simulink model "ControladoresLibro"  (R2025b)
settings: Solver=VariableStepAuto  StartTime=0.0  StopTime=10.0  RelTol=1e-3
libraries: fl_lib x33, slpidlib x18, nesl_utility x18, ee_lib x6
settings Model: Creator=Usuario  LastModifiedBy=Usuario

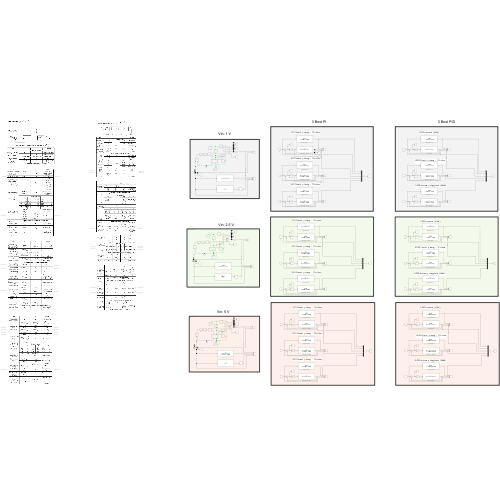
[thumbnail: Simulink's stored preview of the top-level diagram]
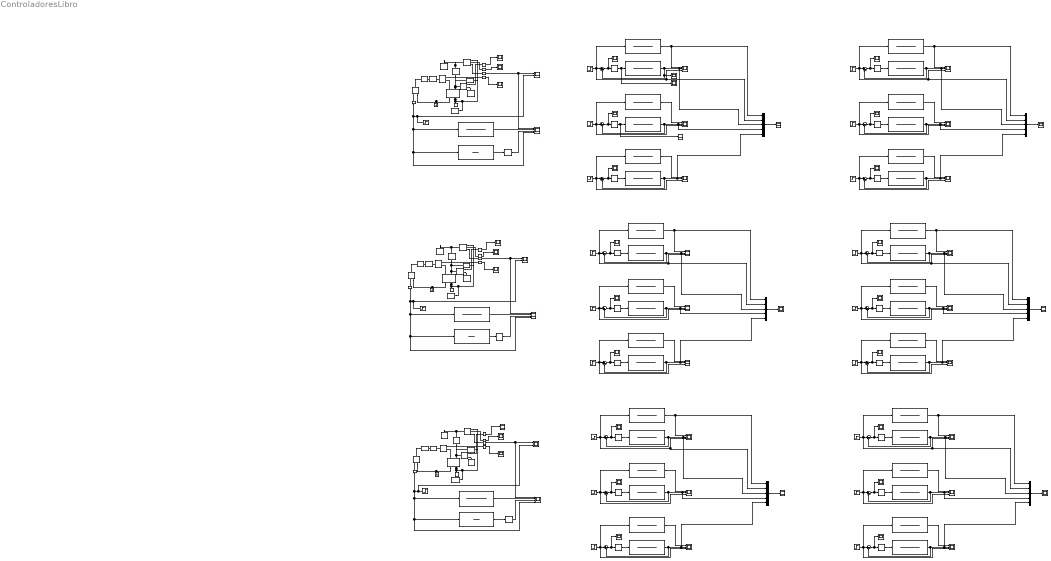
== system ControladoresLibro ==
  note: Voltaje Entrada 1V
  note: --------->
  note: thetha_l
  note: Vin
  note: --------->
  note: Ia
  note: Voltaje Entrada 5V
  note: Vin
  note: thetha_l
  note: Ia
  note: Vin
  note: --------->
  note: Ia
  note: --------->
  note: 1-PI Cluett y Wang - TCL=6tm
  note: <---------
  note: --------->
  note: <---------
  note: 3-PI Cluett y Wang - TCL=4tm
  note: 2-PID Cluett y Wang - TCL=6tm
  note: <---------
  note: thetha_l
  note: 2-PID Cluett y Wang - TCL=6tm
  note: 2-PID Cluett y Wang - TCL=6tm
  note: --------->
  note: 1-PID Leonard (1994)
  note: 3 Best PID
  note: <---------
  note: Vin: 2.5 V
  note: <---------
  note: --------->
  note: 3-PI Cluett y Wang - TCL=4tm
  note: <---------
  note: <---------
  note: <---------
  note: <---------
  note: <---------
  note: --------->
  note: 3-PI Cluett y Wang - TCL=4tm
  note: --------->
  note: 3-PID Astrom y Hagglund (2006)
  note: 2-PI Cluett y Wang - TCL=5tm
  note: --------->
  note: 2-PI Cluett y Wang - TCL=5tm
  note: <---------
  note: 3 Best PI
  note: --------->
  note: 1-PID Leonard (1994)
  note: <---------
  note: 3-PID Astrom y Hagglund (2006)
  note: 2-PI Cluett y Wang - TCL=5tm
  note: Vin: 5 V
  note: 1-PI Cluett y Wang - TCL=6tm
  note: <---------
  note: <---------
  note: --------->
  note: 1-PID Leonard (1994)
  note: --------->
  note: Vin: 1 V
  note: 3-PID Astrom y Hagglund (2006)
  note: <---------
  note: <---------
  note: <---------
  note: <---------
  note: --------->
  note: --------->
  note: 1-PI Cluett y Wang - TCL=6tm
  note: --------->
  note: --------->
  note: Voltaje Entrada 2.5V
  Astrom y Hagglund : TransferFcn  Numerator=[33792]  Denominator=[1 2500 55822 0]
  Astrom y Hagglund1 : TransferFcn  Numerator=[33792]  Denominator=[1 2500 55822 0]
  Astrom y Hagglund2 : TransferFcn  Numerator=[33792]  Denominator=[1 2500 55822 0]
  Cluett y Wang - TCL=4tm : TransferFcn  Numerator=[33792]  Denominator=[1 2500 55822 0]
  Cluett y Wang - TCL=4tm1 : TransferFcn  Numerator=[33792]  Denominator=[1 2500 55822 0]
  Cluett y Wang - TCL=4tm2 : TransferFcn  Numerator=[33792]  Denominator=[1 2500 55822 0]
  Cluett y Wang - TCL=5tm : TransferFcn  Numerator=[33792]  Denominator=[1 2500 55822 0]
  Cluett y Wang - TCL=5tm1 : TransferFcn  Numerator=[33792]  Denominator=[1 2500 55822 0]
  Cluett y Wang - TCL=5tm2 : TransferFcn  Numerator=[33792]  Denominator=[1 2500 55822 0]
  Cluett y Wang - TCL=6tm{,1..5} (6 alike) : TransferFcn  Numerator=[33792]  Denominator=[1 2500 55822 0]
  Controlled Voltage Source : fl_lib/Electrical/Electrical Sources/Controlled Voltage Source
  Controlled Voltage Source1 : fl_lib/Electrical/Electrical Sources/Controlled Voltage Source
  Controlled Voltage Source2 : fl_lib/Electrical/Electrical Sources/Controlled Voltage Source
  Current Sensor : fl_lib/Electrical/Electrical Sensors/Current Sensor
  Current Sensor1 : fl_lib/Electrical/Electrical Sensors/Current Sensor
  Current Sensor2 : fl_lib/Electrical/Electrical Sensors/Current Sensor
  Dm : fl_lib/Mechanical/Rotational Elements/Rotational Damper  D=2.5e-7 N*m*s/rad  w_specify=off  w_priority=None  w=0 rad/s  w_nominal_specify=off  w_nominal_value=1  w_nominal_unit=rad/s  t_specify=off  t_priority=None  t=0 N*m  t_nominal_specify=off  t_nominal_value=1  t_nominal_unit=N*m
  Dm1 : fl_lib/Mechanical/Rotational Elements/Rotational Damper  D=2.5e-7 N*m*s/rad  w_specify=off  w_priority=None  w=0 rad/s  w_nominal_specify=off  w_nominal_value=1  w_nominal_unit=rad/s  t_specify=off  t_priority=None  t=0 N*m  t_nominal_specify=off  t_nominal_value=1  t_nominal_unit=N*m
  Dm2 : fl_lib/Mechanical/Rotational Elements/Rotational Damper  D=2.5e-7 N*m*s/rad  w_specify=off  w_priority=None  w=0 rad/s  w_nominal_specify=off  w_nominal_value=1  w_nominal_unit=rad/s  t_specify=off  t_priority=None  t=0 N*m  t_nominal_specify=off  t_nominal_value=1  t_nominal_unit=N*m
  Electrical Reference : fl_lib/Electrical/Electrical Elements/Electrical Reference
  Electrical Reference1 : fl_lib/Electrical/Electrical Elements/Electrical Reference
  Electrical Reference2 : fl_lib/Electrical/Electrical Elements/Electrical Reference
  Gear Box : fl_lib/Mechanical/Mechanisms/Gear Box  ratio=1/275.6923  t_in_specify=off  t_in_priority=None  t_in=0 N*m  t_in_nominal_specify=off  t_in_nominal_value=1  t_in_nominal_unit=N*m  t_out_specify=off  t_out_priority=None  t_out=0 N*m  t_out_nominal_specify=off  t_out_nominal_value=1  t_out_nominal_unit=N*m
  Gear Box1 : fl_lib/Mechanical/Mechanisms/Gear Box  ratio=1/275.6923  t_in_specify=off  t_in_priority=None  t_in=0 N*m  t_in_nominal_specify=off  t_in_nominal_value=1  t_in_nominal_unit=N*m  t_out_specify=off  t_out_priority=None  t_out=0 N*m  t_out_nominal_specify=off  t_out_nominal_value=1  t_out_nominal_unit=N*m
  Gear Box2 : fl_lib/Mechanical/Mechanisms/Gear Box  ratio=1/275.6923  t_in_specify=off  t_in_priority=None  t_in=0 N*m  t_in_nominal_specify=off  t_in_nominal_value=1  t_in_nominal_unit=N*m  t_out_specify=off  t_out_priority=None  t_out=0 N*m  t_out_nominal_specify=off  t_out_nominal_value=1  t_out_nominal_unit=N*m
  Ideal Rotational Motion Sensor : fl_lib/Mechanical/Mechanical Sensors/Ideal Rotational Motion Sensor  reference=foundation.enum.MeasurementReference.difference  acceleration_port=false  velocity_port=true  position_port=true  wrap_angle=false  offset=0 rad
  Ideal Rotational Motion Sensor1 : fl_lib/Mechanical/Mechanical Sensors/Ideal Rotational Motion Sensor  reference=foundation.enum.MeasurementReference.difference  acceleration_port=false  velocity_port=true  position_port=true  wrap_angle=false  offset=0 rad
  Ideal Rotational Motion Sensor2 : fl_lib/Mechanical/Mechanical Sensors/Ideal Rotational Motion Sensor  reference=foundation.enum.MeasurementReference.difference  acceleration_port=false  velocity_port=true  position_port=true  wrap_angle=false  offset=0 rad
  Ideal Torque Sensor1 : fl_lib/Mechanical/Mechanical Sensors/Ideal Torque Sensor
  Ideal Torque Sensor2 : fl_lib/Mechanical/Mechanical Sensors/Ideal Torque Sensor
  Ideal Torque Sensor3 : fl_lib/Mechanical/Mechanical Sensors/Ideal Torque Sensor
  In1 : Step  SampleTime=0
  In2 : Step  After=2.5  SampleTime=0
  In3 : Step  After=5  SampleTime=0
  In4 : Step  SampleTime=0
  In5 : Step  After=2.5  SampleTime=0
  In6 : Step  After=5  SampleTime=0
  Jl : fl_lib/Mechanical/Rotational Elements/Inertia  inertia=2e-6 kg*m^2  num_ports=foundation.enum.numPorts2.one  w_specify=off  w_priority=High  w=0 rad/s  w_nominal_specify=off  w_nominal_value=1  w_nominal_unit=rad/s  t_specify=off  t_priority=None  t=0 N*m  t_nominal_specify=off  t_nominal_value=1  t_nominal_unit=N*m
  Jl1 : fl_lib/Mechanical/Rotational Elements/Inertia  inertia=2e-6 kg*m^2  num_ports=foundation.enum.numPorts2.one  w_specify=off  w_priority=High  w=0 rad/s  w_nominal_specify=off  w_nominal_value=1  w_nominal_unit=rad/s  t_specify=off  t_priority=None  t=0 N*m  t_nominal_specify=off  t_nominal_value=1  t_nominal_unit=N*m
  Jl2 : fl_lib/Mechanical/Rotational Elements/Inertia  inertia=2e-6 kg*m^2  num_ports=foundation.enum.numPorts2.one  w_specify=off  w_priority=High  w=0 rad/s  w_nominal_specify=off  w_nominal_value=1  w_nominal_unit=rad/s  t_specify=off  t_priority=None  t=0 N*m  t_nominal_specify=off  t_nominal_value=1  t_nominal_unit=N*m
  Jm : fl_lib/Mechanical/Rotational Elements/Inertia  inertia=6.3173e-7 kg*m^2  num_ports=foundation.enum.numPorts2.one  w_specify=off  w_priority=High  w=0 rad/s  w_nominal_specify=off  w_nominal_value=1  w_nominal_unit=rad/s  t_specify=off  t_priority=None  t=0 N*m  t_nominal_specify=off  t_nominal_value=1  t_nominal_unit=N*m
  Jm1 : fl_lib/Mechanical/Rotational Elements/Inertia  inertia=6.3173e-7 kg*m^2  num_ports=foundation.enum.numPorts2.one  w_specify=off  w_priority=High  w=0 rad/s  w_nominal_specify=off  w_nominal_value=1  w_nominal_unit=rad/s  t_specify=off  t_priority=None  t=0 N*m  t_nominal_specify=off  t_nominal_value=1  t_nominal_unit=N*m
  Jm2 : fl_lib/Mechanical/Rotational Elements/Inertia  inertia=6.3173e-7 kg*m^2  num_ports=foundation.enum.numPorts2.one  w_specify=off  w_priority=High  w=0 rad/s  w_nominal_specify=off  w_nominal_value=1  w_nominal_unit=rad/s  t_specify=off  t_priority=None  t=0 N*m  t_nominal_specify=off  t_nominal_value=1  t_nominal_unit=N*m
  L : ee_lib/Passive/Inductor  l=1 mH  enable_L_tol=ee.enum.toleranceApplication.none  L_tol=20  tol_distribution=ee.enum.toleranceDistribution.uniform  nSigma=4  r=0 Ohm  g=0 1/Ohm  enable_operating_limits=ee.enum.enable.no  operating_limit_action=ee.enum.passive.reportOpLim.warn  max_working_current=1 A  power_rating=1 W  i_L_specify=off  i_L_priority=High  i_L=0 A  i_L_nominal_specify=off  i_L_nominal_value=1  i_L_nominal_unit=A
  L1 : ee_lib/Passive/Inductor  l=1 mH  enable_L_tol=ee.enum.toleranceApplication.none  L_tol=20  tol_distribution=ee.enum.toleranceDistribution.uniform  nSigma=4  r=0 Ohm  g=0 1/Ohm  enable_operating_limits=ee.enum.enable.no  operating_limit_action=ee.enum.passive.reportOpLim.warn  max_working_current=1 A  power_rating=1 W  i_L_specify=off  i_L_priority=High  i_L=0 A  i_L_nominal_specify=off  i_L_nominal_value=1  i_L_nominal_unit=A
  L2 : ee_lib/Passive/Inductor  l=1 mH  enable_L_tol=ee.enum.toleranceApplication.none  L_tol=20  tol_distribution=ee.enum.toleranceDistribution.uniform  nSigma=4  r=0 Ohm  g=0 1/Ohm  enable_operating_limits=ee.enum.enable.no  operating_limit_action=ee.enum.passive.reportOpLim.warn  max_working_current=1 A  power_rating=1 W  i_L_specify=off  i_L_priority=High  i_L=0 A  i_L_nominal_specify=off  i_L_nominal_value=1  i_L_nominal_unit=A
  Leonard (1994) : TransferFcn  Numerator=[33792]  Denominator=[1 2500 55822 0]
  Leonard (1994)1 : TransferFcn  Numerator=[33792]  Denominator=[1 2500 55822 0]
  Leonard (1994)2 : TransferFcn  Numerator=[33792]  Denominator=[1 2500 55822 0]
  Mechanical Rotational Reference : fl_lib/Mechanical/Rotational Elements/Mechanical Rotational Reference
  Mechanical Rotational Reference1 : fl_lib/Mechanical/Rotational Elements/Mechanical Rotational Reference
  Mechanical Rotational Reference2 : fl_lib/Mechanical/Rotational Elements/Mechanical Rotational Reference
  Mux{1..6} (6 alike) : Mux  Inputs=5
  Original Function {1..18} (18 alike) : TransferFcn  Numerator=[33792]  Denominator=[1 2500 55822 0]
  PID Controller{7,10,12,15,17} (5 alike) : slpidlib/PID Controller  Controller=PI  Form=Parallel  TimeDomain=Continuous-time  UseExternalTs=off  SampleTime=-1  IntegratorMethod=Forward Euler  FilterMethod=Forward Euler  ControllerParametersSource=internal  P=11.1080  I=21.4441  UseKiTs=off  D=1.316  UseExternalDerivativeSource=off  N=100  UseFilter=on  TunerSelectOption=Transfer Function Based (PID Tuner App)  InitialConditionSource=internal  InitialConditionForIntegrator=0  InitialConditionForFilter=0  DifferentiatorICPrevScaledInput=0  ExternalReset=none  TrackingMode=off  Kt=1  LimitOutput=off  SatLimitsSource=internal  UpperSaturationLimit=inf  LowerSaturationLimit=-inf  LinearizeAsGain=on  AntiWindupMode=none  Kb=1  LimitIntegrator=off  UpperIntegratorSaturationLimit=inf  LowerIntegratorSaturationLimit=-inf  POutMin=[]  POutMax=[]  IOutMin=[]  IOutMax=[]  DOutMin=[]  DOutMax=[]  NOutMin=[]  NOutMax=[]  SumOutMin=[]  SumOutMax=[]  SaturationOutMin=[]  SaturationOutMax=[]  PParamMin=[]  PParamMax=[]  IParamMin=[]  IParamMax=[]  DParamMin=[]  DParamMax=[]  NParamMin=[]  NParamMax=[]  KbParamMin=[]  KbParamMax=[]  KtParamMin=[]  KtParamMax=[]  KbOutMin=[]  KbOutMax=[]  KtOutMin=[]  KtOutMax=[]  IntegratorOutMin=[]  IntegratorOutMax=[]  FilterOutMin=[]  FilterOutMax=[]  SumI1OutMin=[]  SumI1OutMax=[]  SumI2OutMin=[]  SumI2OutMax=[]  SumI3OutMin=[]  SumI3OutMax=[]  SumI4OutMin=[]  SumI4OutMax=[]  SumDOutMin=[]  SumDOutMax=[]  DifferentiatorOutMin=[]  DifferentiatorOutMax=[]  FilterDiffOutCoefMin=[]  FilterDiffOutCoefMax=[]  ReciprocalOutMin=[]  ReciprocalOutMax=[]  SumDenOutMin=[]  SumDenOutMax=[]  SumNumOutMin=[]  SumNumOutMax=[]  DivideOutMin=[]  DivideOutMax=[]  UdiffTsProdOutMin=[]  UdiffTsProdOutMax=[]  NTsProdOutMin=[]  NTsProdOutMax=[]  UintegralTsProdOutMin=[]  UintegralTsProdOutMax=[]  UngainTsProdOutMin=[]  UngainTsProdOutMax=[]  ClampingZeroOutDataTypeStr=Inherit: Inherit via back propagation  ClampingZeroOutMin=[]  ClampingZeroOutMax=[]  FilterDenConstantOutDataTypeStr=Inherit: Inherit via back propagation  FilterDenConstantOutMin=[]  FilterDenConstantOutMax=[]  PCopyOutDataTypeStr=Inherit: Inherit via back propagation  PCopyOutMin=[]  PCopyOutMax=[]  NCopyOutDataTypeStr=Inherit: Inherit via back propagation  NCopyOutMin=[]  NCopyOutMax=[]  IntegratorContinuousStateAttributes=''  IntegratorStateMustResolveToSignalObject=off  IntegratorRTWStateStorageClass=Auto  FilterContinuousStateAttributes=''  FilterStateMustResolveToSignalObject=off  FilterRTWStateStorageClass=Auto  ParallelPVariant=InternalParameters  IdealPVariant=Disabled  IVariant=InternalParameters  DVariant=Disabled  IntegratorVariant=Continuous  SatVariant=Disabled  AWVariant=Passthrough  PCopyVariant=Disabled  TRVariant=Disabled  FdbkBlocksVariant=Forward  IdealPFdbkVariant=Disabled  SatFdbkVariant=Disabled  DerivativeFilterVariant=Disabled  NVariant=Disabled  NCopyVariant=Disabled_SignalSpec  FilterICVariant=Disabled  IntegratorICVariant=InternalICs  ExternalResetVariant=Disabled  TRSumVariant=Passthrough  SumFdbkVariant=Disabled  SumVariant=Sum_PI  TsampFilterVariant=InternalTs  TsampNgainVariant=Passthrough  TsampIntegralVariant=Disabled_SignalSpec  ExternalSaturationOutDataTypeStr=Inherit: Same as second input  DerivativeSourceVariant=Disabled  PreIntVariant=InternalPreInt
  PID Controller{8,11,13,16,18} (5 alike) : slpidlib/PID Controller  Controller=PI  Form=Parallel  TimeDomain=Continuous-time  UseExternalTs=off  SampleTime=-1  IntegratorMethod=Forward Euler  FilterMethod=Forward Euler  ControllerParametersSource=internal  P=13.2561  I=31.0787  UseKiTs=off  D=1.316  UseExternalDerivativeSource=off  N=100  UseFilter=on  TunerSelectOption=Transfer Function Based (PID Tuner App)  InitialConditionSource=internal  InitialConditionForIntegrator=0  InitialConditionForFilter=0  DifferentiatorICPrevScaledInput=0  ExternalReset=none  TrackingMode=off  Kt=1  LimitOutput=off  SatLimitsSource=internal  UpperSaturationLimit=inf  LowerSaturationLimit=-inf  LinearizeAsGain=on  AntiWindupMode=none  Kb=1  LimitIntegrator=off  UpperIntegratorSaturationLimit=inf  LowerIntegratorSaturationLimit=-inf  POutMin=[]  POutMax=[]  IOutMin=[]  IOutMax=[]  DOutMin=[]  DOutMax=[]  NOutMin=[]  NOutMax=[]  SumOutMin=[]  SumOutMax=[]  SaturationOutMin=[]  SaturationOutMax=[]  PParamMin=[]  PParamMax=[]  IParamMin=[]  IParamMax=[]  DParamMin=[]  DParamMax=[]  NParamMin=[]  NParamMax=[]  KbParamMin=[]  KbParamMax=[]  KtParamMin=[]  KtParamMax=[]  KbOutMin=[]  KbOutMax=[]  KtOutMin=[]  KtOutMax=[]  IntegratorOutMin=[]  IntegratorOutMax=[]  FilterOutMin=[]  FilterOutMax=[]  SumI1OutMin=[]  SumI1OutMax=[]  SumI2OutMin=[]  SumI2OutMax=[]  SumI3OutMin=[]  SumI3OutMax=[]  SumI4OutMin=[]  SumI4OutMax=[]  SumDOutMin=[]  SumDOutMax=[]  DifferentiatorOutMin=[]  DifferentiatorOutMax=[]  FilterDiffOutCoefMin=[]  FilterDiffOutCoefMax=[]  ReciprocalOutMin=[]  ReciprocalOutMax=[]  SumDenOutMin=[]  SumDenOutMax=[]  SumNumOutMin=[]  SumNumOutMax=[]  DivideOutMin=[]  DivideOutMax=[]  UdiffTsProdOutMin=[]  UdiffTsProdOutMax=[]  NTsProdOutMin=[]  NTsProdOutMax=[]  UintegralTsProdOutMin=[]  UintegralTsProdOutMax=[]  UngainTsProdOutMin=[]  UngainTsProdOutMax=[]  ClampingZeroOutDataTypeStr=Inherit: Inherit via back propagation  ClampingZeroOutMin=[]  ClampingZeroOutMax=[]  FilterDenConstantOutDataTypeStr=Inherit: Inherit via back propagation  FilterDenConstantOutMin=[]  FilterDenConstantOutMax=[]  PCopyOutDataTypeStr=Inherit: Inherit via back propagation  PCopyOutMin=[]  PCopyOutMax=[]  NCopyOutDataTypeStr=Inherit: Inherit via back propagation  NCopyOutMin=[]  NCopyOutMax=[]  IntegratorContinuousStateAttributes=''  IntegratorStateMustResolveToSignalObject=off  IntegratorRTWStateStorageClass=Auto  FilterContinuousStateAttributes=''  FilterStateMustResolveToSignalObject=off  FilterRTWStateStorageClass=Auto  ParallelPVariant=InternalParameters  IdealPVariant=Disabled  IVariant=InternalParameters  DVariant=Disabled  IntegratorVariant=Continuous  SatVariant=Disabled  AWVariant=Passthrough  PCopyVariant=Disabled  TRVariant=Disabled  FdbkBlocksVariant=Forward  IdealPFdbkVariant=Disabled  SatFdbkVariant=Disabled  DerivativeFilterVariant=Disabled  NVariant=Disabled  NCopyVariant=Disabled_SignalSpec  FilterICVariant=Disabled  IntegratorICVariant=InternalICs  ExternalResetVariant=Disabled  TRSumVariant=Passthrough  SumFdbkVariant=Disabled  SumVariant=Sum_PI  TsampFilterVariant=InternalTs  TsampNgainVariant=Passthrough  TsampIntegralVariant=Disabled_SignalSpec  ExternalSaturationOutDataTypeStr=Inherit: Same as second input  DerivativeSourceVariant=Disabled  PreIntVariant=InternalPreInt
  PID Controller{6,9,14,19,23} (5 alike) : slpidlib/PID Controller  Controller=PI  Form=Parallel  TimeDomain=Continuous-time  UseExternalTs=off  SampleTime=-1  IntegratorMethod=Forward Euler  FilterMethod=Forward Euler  ControllerParametersSource=internal  P=9.5711  I=15.6962  UseKiTs=off  D=1.316  UseExternalDerivativeSource=off  N=100  UseFilter=on  TunerSelectOption=Transfer Function Based (PID Tuner App)  InitialConditionSource=internal  InitialConditionForIntegrator=0  InitialConditionForFilter=0  DifferentiatorICPrevScaledInput=0  ExternalReset=none  TrackingMode=off  Kt=1  LimitOutput=off  SatLimitsSource=internal  UpperSaturationLimit=inf  LowerSaturationLimit=-inf  LinearizeAsGain=on  AntiWindupMode=none  Kb=1  LimitIntegrator=off  UpperIntegratorSaturationLimit=inf  LowerIntegratorSaturationLimit=-inf  POutMin=[]  POutMax=[]  IOutMin=[]  IOutMax=[]  DOutMin=[]  DOutMax=[]  NOutMin=[]  NOutMax=[]  SumOutMin=[]  SumOutMax=[]  SaturationOutMin=[]  SaturationOutMax=[]  PParamMin=[]  PParamMax=[]  IParamMin=[]  IParamMax=[]  DParamMin=[]  DParamMax=[]  NParamMin=[]  NParamMax=[]  KbParamMin=[]  KbParamMax=[]  KtParamMin=[]  KtParamMax=[]  KbOutMin=[]  KbOutMax=[]  KtOutMin=[]  KtOutMax=[]  IntegratorOutMin=[]  IntegratorOutMax=[]  FilterOutMin=[]  FilterOutMax=[]  SumI1OutMin=[]  SumI1OutMax=[]  SumI2OutMin=[]  SumI2OutMax=[]  SumI3OutMin=[]  SumI3OutMax=[]  SumI4OutMin=[]  SumI4OutMax=[]  SumDOutMin=[]  SumDOutMax=[]  DifferentiatorOutMin=[]  DifferentiatorOutMax=[]  FilterDiffOutCoefMin=[]  FilterDiffOutCoefMax=[]  ReciprocalOutMin=[]  ReciprocalOutMax=[]  SumDenOutMin=[]  SumDenOutMax=[]  SumNumOutMin=[]  SumNumOutMax=[]  DivideOutMin=[]  DivideOutMax=[]  UdiffTsProdOutMin=[]  UdiffTsProdOutMax=[]  NTsProdOutMin=[]  NTsProdOutMax=[]  UintegralTsProdOutMin=[]  UintegralTsProdOutMax=[]  UngainTsProdOutMin=[]  UngainTsProdOutMax=[]  ClampingZeroOutDataTypeStr=Inherit: Inherit via back propagation  ClampingZeroOutMin=[]  ClampingZeroOutMax=[]  FilterDenConstantOutDataTypeStr=Inherit: Inherit via back propagation  FilterDenConstantOutMin=[]  FilterDenConstantOutMax=[]  PCopyOutDataTypeStr=Inherit: Inherit via back propagation  PCopyOutMin=[]  PCopyOutMax=[]  NCopyOutDataTypeStr=Inherit: Inherit via back propagation  NCopyOutMin=[]  NCopyOutMax=[]  IntegratorContinuousStateAttributes=''  IntegratorStateMustResolveToSignalObject=off  IntegratorRTWStateStorageClass=Auto  FilterContinuousStateAttributes=''  FilterStateMustResolveToSignalObject=off  FilterRTWStateStorageClass=Auto  ParallelPVariant=InternalParameters  IdealPVariant=Disabled  IVariant=InternalParameters  DVariant=Disabled  IntegratorVariant=Continuous  SatVariant=Disabled  AWVariant=Passthrough  PCopyVariant=Disabled  TRVariant=Disabled  FdbkBlocksVariant=Forward  IdealPFdbkVariant=Disabled  SatFdbkVariant=Disabled  DerivativeFilterVariant=Disabled  NVariant=Disabled  NCopyVariant=Disabled_SignalSpec  FilterICVariant=Disabled  IntegratorICVariant=InternalICs  ExternalResetVariant=Disabled  TRSumVariant=Passthrough  SumFdbkVariant=Disabled  SumVariant=Sum_PI  TsampFilterVariant=InternalTs  TsampNgainVariant=Passthrough  TsampIntegralVariant=Disabled_SignalSpec  ExternalSaturationOutDataTypeStr=Inherit: Same as second input  DerivativeSourceVariant=Disabled  PreIntVariant=InternalPreInt
  PID Controller20 : slpidlib/PID Controller  Controller=PID  Form=Parallel  TimeDomain=Continuous-time  UseExternalTs=off  SampleTime=-1  IntegratorMethod=Forward Euler  FilterMethod=Forward Euler  ControllerParametersSource=internal  P=26.1447  I=46.1855  UseKiTs=off  D=0.4974  UseExternalDerivativeSource=off  N=100  UseFilter=on  TunerSelectOption=Transfer Function Based (PID Tuner App)  InitialConditionSource=internal  InitialConditionForIntegrator=0  InitialConditionForFilter=0  DifferentiatorICPrevScaledInput=0  ExternalReset=none  TrackingMode=off  Kt=1  LimitOutput=off  SatLimitsSource=internal  UpperSaturationLimit=inf  LowerSaturationLimit=-inf  LinearizeAsGain=on  AntiWindupMode=none  Kb=1  LimitIntegrator=off  UpperIntegratorSaturationLimit=inf  LowerIntegratorSaturationLimit=-inf  POutMin=[]  POutMax=[]  IOutMin=[]  IOutMax=[]  DOutMin=[]  DOutMax=[]  NOutMin=[]  NOutMax=[]  SumOutMin=[]  SumOutMax=[]  SaturationOutMin=[]  SaturationOutMax=[]  PParamMin=[]  PParamMax=[]  IParamMin=[]  IParamMax=[]  DParamMin=[]  DParamMax=[]  NParamMin=[]  NParamMax=[]  KbParamMin=[]  KbParamMax=[]  KtParamMin=[]  KtParamMax=[]  KbOutMin=[]  KbOutMax=[]  KtOutMin=[]  KtOutMax=[]  IntegratorOutMin=[]  IntegratorOutMax=[]  FilterOutMin=[]  FilterOutMax=[]  SumI1OutMin=[]  SumI1OutMax=[]  SumI2OutMin=[]  SumI2OutMax=[]  SumI3OutMin=[]  SumI3OutMax=[]  SumI4OutMin=[]  SumI4OutMax=[]  SumDOutMin=[]  SumDOutMax=[]  DifferentiatorOutMin=[]  DifferentiatorOutMax=[]  FilterDiffOutCoefMin=[]  FilterDiffOutCoefMax=[]  ReciprocalOutMin=[]  ReciprocalOutMax=[]  SumDenOutMin=[]  SumDenOutMax=[]  SumNumOutMin=[]  SumNumOutMax=[]  DivideOutMin=[]  DivideOutMax=[]  UdiffTsProdOutMin=[]  UdiffTsProdOutMax=[]  NTsProdOutMin=[]  NTsProdOutMax=[]  UintegralTsProdOutMin=[]  UintegralTsProdOutMax=[]  UngainTsProdOutMin=[]  UngainTsProdOutMax=[]  ClampingZeroOutDataTypeStr=Inherit: Inherit via back propagation  ClampingZeroOutMin=[]  ClampingZeroOutMax=[]  FilterDenConstantOutDataTypeStr=Inherit: Inherit via back propagation  FilterDenConstantOutMin=[]  FilterDenConstantOutMax=[]  PCopyOutDataTypeStr=Inherit: Inherit via back propagation  PCopyOutMin=[]  PCopyOutMax=[]  NCopyOutDataTypeStr=Inherit: Inherit via back propagation  NCopyOutMin=[]  NCopyOutMax=[]  IntegratorContinuousStateAttributes=''  IntegratorStateMustResolveToSignalObject=off  IntegratorRTWStateStorageClass=Auto  FilterContinuousStateAttributes=''  FilterStateMustResolveToSignalObject=off  FilterRTWStateStorageClass=Auto  ParallelPVariant=InternalParameters  IdealPVariant=Disabled  IVariant=InternalParameters  DVariant=InternalParameters  IntegratorVariant=Continuous  SatVariant=Disabled  AWVariant=Passthrough  PCopyVariant=Disabled  TRVariant=Disabled  FdbkBlocksVariant=Forward  IdealPFdbkVariant=Disabled  SatFdbkVariant=Disabled  DerivativeFilterVariant=ContFilter  NVariant=InternalParameters  NCopyVariant=Disabled  FilterICVariant=InternalICsFilter  IntegratorICVariant=InternalICs  ExternalResetVariant=Disabled  TRSumVariant=Passthrough  SumFdbkVariant=Disabled  SumVariant=Sum_PID  TsampFilterVariant=InternalTs  TsampNgainVariant=Passthrough  TsampIntegralVariant=Disabled_SignalSpec  ExternalSaturationOutDataTypeStr=Inherit: Same as second input  DerivativeSourceVariant=ErrorSignal  PreIntVariant=InternalPreInt
  PID Controller21 : slpidlib/PID Controller  Controller=PID  Form=Parallel  TimeDomain=Continuous-time  UseExternalTs=off  SampleTime=-1  IntegratorMethod=Forward Euler  FilterMethod=Forward Euler  ControllerParametersSource=internal  P=9.5711  I=15.6962  UseKiTs=off  D=0.0564  UseExternalDerivativeSource=off  N=100  UseFilter=on  TunerSelectOption=Transfer Function Based (PID Tuner App)  InitialConditionSource=internal  InitialConditionForIntegrator=0  InitialConditionForFilter=0  DifferentiatorICPrevScaledInput=0  ExternalReset=none  TrackingMode=off  Kt=1  LimitOutput=off  SatLimitsSource=internal  UpperSaturationLimit=inf  LowerSaturationLimit=-inf  LinearizeAsGain=on  AntiWindupMode=none  Kb=1  LimitIntegrator=off  UpperIntegratorSaturationLimit=inf  LowerIntegratorSaturationLimit=-inf  POutMin=[]  POutMax=[]  IOutMin=[]  IOutMax=[]  DOutMin=[]  DOutMax=[]  NOutMin=[]  NOutMax=[]  SumOutMin=[]  SumOutMax=[]  SaturationOutMin=[]  SaturationOutMax=[]  PParamMin=[]  PParamMax=[]  IParamMin=[]  IParamMax=[]  DParamMin=[]  DParamMax=[]  NParamMin=[]  NParamMax=[]  KbParamMin=[]  KbParamMax=[]  KtParamMin=[]  KtParamMax=[]  KbOutMin=[]  KbOutMax=[]  KtOutMin=[]  KtOutMax=[]  IntegratorOutMin=[]  IntegratorOutMax=[]  FilterOutMin=[]  FilterOutMax=[]  SumI1OutMin=[]  SumI1OutMax=[]  SumI2OutMin=[]  SumI2OutMax=[]  SumI3OutMin=[]  SumI3OutMax=[]  SumI4OutMin=[]  SumI4OutMax=[]  SumDOutMin=[]  SumDOutMax=[]  DifferentiatorOutMin=[]  DifferentiatorOutMax=[]  FilterDiffOutCoefMin=[]  FilterDiffOutCoefMax=[]  ReciprocalOutMin=[]  ReciprocalOutMax=[]  SumDenOutMin=[]  SumDenOutMax=[]  SumNumOutMin=[]  SumNumOutMax=[]  DivideOutMin=[]  DivideOutMax=[]  UdiffTsProdOutMin=[]  UdiffTsProdOutMax=[]  NTsProdOutMin=[]  NTsProdOutMax=[]  UintegralTsProdOutMin=[]  UintegralTsProdOutMax=[]  UngainTsProdOutMin=[]  UngainTsProdOutMax=[]  ClampingZeroOutDataTypeStr=Inherit: Inherit via back propagation  ClampingZeroOutMin=[]  ClampingZeroOutMax=[]  FilterDenConstantOutDataTypeStr=Inherit: Inherit via back propagation  FilterDenConstantOutMin=[]  FilterDenConstantOutMax=[]  PCopyOutDataTypeStr=Inherit: Inherit via back propagation  PCopyOutMin=[]  PCopyOutMax=[]  NCopyOutDataTypeStr=Inherit: Inherit via back propagation  NCopyOutMin=[]  NCopyOutMax=[]  IntegratorContinuousStateAttributes=''  IntegratorStateMustResolveToSignalObject=off  IntegratorRTWStateStorageClass=Auto  FilterContinuousStateAttributes=''  FilterStateMustResolveToSignalObject=off  FilterRTWStateStorageClass=Auto  ParallelPVariant=InternalParameters  IdealPVariant=Disabled  IVariant=InternalParameters  DVariant=InternalParameters  IntegratorVariant=Continuous  SatVariant=Disabled  AWVariant=Passthrough  PCopyVariant=Disabled  TRVariant=Disabled  FdbkBlocksVariant=Forward  IdealPFdbkVariant=Disabled  SatFdbkVariant=Disabled  DerivativeFilterVariant=ContFilter  NVariant=InternalParameters  NCopyVariant=Disabled  FilterICVariant=InternalICsFilter  IntegratorICVariant=InternalICs  ExternalResetVariant=Disabled  TRSumVariant=Passthrough  SumFdbkVariant=Disabled  SumVariant=Sum_PID  TsampFilterVariant=InternalTs  TsampNgainVariant=Passthrough  TsampIntegralVariant=Disabled_SignalSpec  ExternalSaturationOutDataTypeStr=Inherit: Same as second input  DerivativeSourceVariant=ErrorSignal  PreIntVariant=InternalPreInt
  PID Controller22 : slpidlib/PID Controller  Controller=PID  Form=Parallel  TimeDomain=Continuous-time  UseExternalTs=off  SampleTime=-1  IntegratorMethod=Forward Euler  FilterMethod=Forward Euler  ControllerParametersSource=internal  P=15.8988  I=42.8309  UseKiTs=off  D=0.3689  UseExternalDerivativeSource=off  N=100  UseFilter=on  TunerSelectOption=Transfer Function Based (PID Tuner App)  InitialConditionSource=internal  InitialConditionForIntegrator=0  InitialConditionForFilter=0  DifferentiatorICPrevScaledInput=0  ExternalReset=none  TrackingMode=off  Kt=1  LimitOutput=off  SatLimitsSource=internal  UpperSaturationLimit=inf  LowerSaturationLimit=-inf  LinearizeAsGain=on  AntiWindupMode=none  Kb=1  LimitIntegrator=off  UpperIntegratorSaturationLimit=inf  LowerIntegratorSaturationLimit=-inf  POutMin=[]  POutMax=[]  IOutMin=[]  IOutMax=[]  DOutMin=[]  DOutMax=[]  NOutMin=[]  NOutMax=[]  SumOutMin=[]  SumOutMax=[]  SaturationOutMin=[]  SaturationOutMax=[]  PParamMin=[]  PParamMax=[]  IParamMin=[]  IParamMax=[]  DParamMin=[]  DParamMax=[]  NParamMin=[]  NParamMax=[]  KbParamMin=[]  KbParamMax=[]  KtParamMin=[]  KtParamMax=[]  KbOutMin=[]  KbOutMax=[]  KtOutMin=[]  KtOutMax=[]  IntegratorOutMin=[]  IntegratorOutMax=[]  FilterOutMin=[]  FilterOutMax=[]  SumI1OutMin=[]  SumI1OutMax=[]  SumI2OutMin=[]  SumI2OutMax=[]  SumI3OutMin=[]  SumI3OutMax=[]  SumI4OutMin=[]  SumI4OutMax=[]  SumDOutMin=[]  SumDOutMax=[]  DifferentiatorOutMin=[]  DifferentiatorOutMax=[]  FilterDiffOutCoefMin=[]  FilterDiffOutCoefMax=[]  ReciprocalOutMin=[]  ReciprocalOutMax=[]  SumDenOutMin=[]  SumDenOutMax=[]  SumNumOutMin=[]  SumNumOutMax=[]  DivideOutMin=[]  DivideOutMax=[]  UdiffTsProdOutMin=[]  UdiffTsProdOutMax=[]  NTsProdOutMin=[]  NTsProdOutMax=[]  UintegralTsProdOutMin=[]  UintegralTsProdOutMax=[]  UngainTsProdOutMin=[]  UngainTsProdOutMax=[]  ClampingZeroOutDataTypeStr=Inherit: Inherit via back propagation  ClampingZeroOutMin=[]  ClampingZeroOutMax=[]  FilterDenConstantOutDataTypeStr=Inherit: Inherit via back propagation  FilterDenConstantOutMin=[]  FilterDenConstantOutMax=[]  PCopyOutDataTypeStr=Inherit: Inherit via back propagation  PCopyOutMin=[]  PCopyOutMax=[]  NCopyOutDataTypeStr=Inherit: Inherit via back propagation  NCopyOutMin=[]  NCopyOutMax=[]  IntegratorContinuousStateAttributes=''  IntegratorStateMustResolveToSignalObject=off  IntegratorRTWStateStorageClass=Auto  FilterContinuousStateAttributes=''  FilterStateMustResolveToSignalObject=off  FilterRTWStateStorageClass=Auto  ParallelPVariant=InternalParameters  IdealPVariant=Disabled  IVariant=InternalParameters  DVariant=InternalParameters  IntegratorVariant=Continuous  SatVariant=Disabled  AWVariant=Passthrough  PCopyVariant=Disabled  TRVariant=Disabled  FdbkBlocksVariant=Forward  IdealPFdbkVariant=Disabled  SatFdbkVariant=Disabled  DerivativeFilterVariant=ContFilter  NVariant=InternalParameters  NCopyVariant=Disabled  FilterICVariant=InternalICsFilter  IntegratorICVariant=InternalICs  ExternalResetVariant=Disabled  TRSumVariant=Passthrough  SumFdbkVariant=Disabled  SumVariant=Sum_PID  TsampFilterVariant=InternalTs  TsampNgainVariant=Passthrough  TsampIntegralVariant=Disabled_SignalSpec  ExternalSaturationOutDataTypeStr=Inherit: Same as second input  DerivativeSourceVariant=ErrorSignal  PreIntVariant=InternalPreInt
  PS-Simulink Converter : nesl_utility/PS-Simulink Converter  PhysicalDomain=network_engine_domain  SubClassName=ps_output  LeftPortType=input  RightPortType=output  PseudoPeriodic=off  Frequencies=[]  VectorFormat=inherit  Unit=rad  AffineConversion=off
  PS-Simulink Converter1 : nesl_utility/PS-Simulink Converter  PhysicalDomain=network_engine_domain  SubClassName=ps_output  LeftPortType=input  RightPortType=output  PseudoPeriodic=off  Frequencies=[]  VectorFormat=inherit  Unit=A  AffineConversion=off
  PS-Simulink Converter{2..3,6..7,10..11} (6 alike) : nesl_utility/PS-Simulink Converter  PhysicalDomain=network_engine_domain  SubClassName=ps_output  LeftPortType=input  RightPortType=output  PseudoPeriodic=off  Frequencies=[]  VectorFormat=inherit  Unit=inherit  AffineConversion=off
  PS-Simulink Converter4 : nesl_utility/PS-Simulink Converter  PhysicalDomain=network_engine_domain  SubClassName=ps_output  LeftPortType=input  RightPortType=output  PseudoPeriodic=off  Frequencies=[]  VectorFormat=inherit  Unit=rad  AffineConversion=off
  PS-Simulink Converter5 : nesl_utility/PS-Simulink Converter  PhysicalDomain=network_engine_domain  SubClassName=ps_output  LeftPortType=input  RightPortType=output  PseudoPeriodic=off  Frequencies=[]  VectorFormat=inherit  Unit=A  AffineConversion=off
  PS-Simulink Converter8 : nesl_utility/PS-Simulink Converter  PhysicalDomain=network_engine_domain  SubClassName=ps_output  LeftPortType=input  RightPortType=output  PseudoPeriodic=off  Frequencies=[]  VectorFormat=inherit  Unit=rad  AffineConversion=off
  PS-Simulink Converter9 : nesl_utility/PS-Simulink Converter  PhysicalDomain=network_engine_domain  SubClassName=ps_output  LeftPortType=input  RightPortType=output  PseudoPeriodic=off  Frequencies=[]  VectorFormat=inherit  Unit=A  AffineConversion=off
  R : ee_lib/Passive/Resistor  R=2.5 Ohm  enable_R_tol=ee.enum.toleranceApplication.none  R_tol=5  tol_distribution=ee.enum.toleranceDistribution.uniform  nSigma=4  enable_operating_limits=ee.enum.enable.no  operating_limit_action=ee.enum.passive.reportOpLim.warn  power_rating=1 W  max_working_voltage=100 V  noise_mode=ee.enum.sources.noise.Disabled  Tdevice=25 degC  sample_time=1e-3 s  repeatability=ee.enum.ic.repeatability.notRepeatable  user_seed=0  auto_seed=3499211588  power_derating_T1=70 degC  power_derating_T2=155 degC  operating_temperature_range_vec=[-50, 150] degC  alpha=3.93e-3 1/K  Tmeas=25 degC  thermal_mass=100 J/K  temperature_specify=off  temperature_priority=High  temperature=298.15 K  temperature_nominal_specify=off  temperature_nominal_value=1  temperature_nominal_unit=K
  R1 : ee_lib/Passive/Resistor  R=2.5 Ohm  enable_R_tol=ee.enum.toleranceApplication.none  R_tol=5  tol_distribution=ee.enum.toleranceDistribution.uniform  nSigma=4  enable_operating_limits=ee.enum.enable.no  operating_limit_action=ee.enum.passive.reportOpLim.warn  power_rating=1 W  max_working_voltage=100 V  noise_mode=ee.enum.sources.noise.Disabled  Tdevice=25 degC  sample_time=1e-3 s  repeatability=ee.enum.ic.repeatability.notRepeatable  user_seed=0  auto_seed=3890346746  power_derating_T1=70 degC  power_derating_T2=155 degC  operating_temperature_range_vec=[-50, 150] degC  alpha=3.93e-3 1/K  Tmeas=25 degC  thermal_mass=100 J/K  temperature_specify=off  temperature_priority=High  temperature=298.15 K  temperature_nominal_specify=off  temperature_nominal_value=1  temperature_nominal_unit=K
  R2 : ee_lib/Passive/Resistor  R=2.5 Ohm  enable_R_tol=ee.enum.toleranceApplication.none  R_tol=5  tol_distribution=ee.enum.toleranceDistribution.uniform  nSigma=4  enable_operating_limits=ee.enum.enable.no  operating_limit_action=ee.enum.passive.reportOpLim.warn  power_rating=1 W  max_working_voltage=100 V  noise_mode=ee.enum.sources.noise.Disabled  Tdevice=25 degC  sample_time=1e-3 s  repeatability=ee.enum.ic.repeatability.notRepeatable  user_seed=0  auto_seed=545404223  power_derating_T1=70 degC  power_derating_T2=155 degC  operating_temperature_range_vec=[-50, 150] degC  alpha=3.93e-3 1/K  Tmeas=25 degC  thermal_mass=100 J/K  temperature_specify=off  temperature_priority=High  temperature=298.15 K  temperature_nominal_specify=off  temperature_nominal_value=1  temperature_nominal_unit=K
  Rotational Electromechanical Converter : fl_lib/Electrical/Electrical Elements/Rotational Electromechanical Converter  K=5.8857e-3 V*s/rad  i_specify=off  i_priority=None  i=0 A  i_nominal_specify=off  i_nominal_value=1  i_nominal_unit=A  v_specify=off  v_priority=None  v=0 V  v_nominal_specify=off  v_nominal_value=1  v_nominal_unit=V  t_specify=off  t_priority=None  t=0 N*m  t_nominal_specify=off  t_nominal_value=1  t_nominal_unit=N*m  w_specify=off  w_priority=None  w=0 rad/s  w_nominal_specify=off  w_nominal_value=1  w_nominal_unit=rad/s
  Rotational Electromechanical Converter1 : fl_lib/Electrical/Electrical Elements/Rotational Electromechanical Converter  K=5.8857e-3 V*s/rad  i_specify=off  i_priority=None  i=0 A  i_nominal_specify=off  i_nominal_value=1  i_nominal_unit=A  v_specify=off  v_priority=None  v=0 V  v_nominal_specify=off  v_nominal_value=1  v_nominal_unit=V  t_specify=off  t_priority=None  t=0 N*m  t_nominal_specify=off  t_nominal_value=1  t_nominal_unit=N*m  w_specify=off  w_priority=None  w=0 rad/s  w_nominal_specify=off  w_nominal_value=1  w_nominal_unit=rad/s
  Rotational Electromechanical Converter2 : fl_lib/Electrical/Electrical Elements/Rotational Electromechanical Converter  K=5.8857e-3 V*s/rad  i_specify=off  i_priority=None  i=0 A  i_nominal_specify=off  i_nominal_value=1  i_nominal_unit=A  v_specify=off  v_priority=None  v=0 V  v_nominal_specify=off  v_nominal_value=1  v_nominal_unit=V  t_specify=off  t_priority=None  t=0 N*m  t_nominal_specify=off  t_nominal_value=1  t_nominal_unit=N*m  w_specify=off  w_priority=None  w=0 rad/s  w_nominal_specify=off  w_nominal_value=1  w_nominal_unit=rad/s
  Scope{1..2,4,18,20,22..23,25,27,29,31,33..34,36,38,40..41,43,45,47..48,50,52,54..55,57,59,61..62,64,66,68..72} (36 alike) : Scope
      Scope18 settings: DataLoggingVariableName=ScopeData18
      Scope2 settings: ActiveDisplayYMinimum=-1  ActiveDisplayYMaximum=1  DataLoggingVariableName=ScopeData2
      Scope20 settings: ActiveDisplayYMinimum=-1  ActiveDisplayYMaximum=1  DataLoggingVariableName=ScopeData20
      Scope22 settings: ActiveDisplayYMinimum=-0.075670313190525529  ActiveDisplayYMaximum=0.68103281871472987  DataLoggingVariableName=ScopeData22
      Scope23 settings: DataLoggingVariableName=ScopeData23
      Scope25 settings: ActiveDisplayYMinimum=-1  ActiveDisplayYMaximum=1  DataLoggingVariableName=ScopeData25
      Scope27 settings: ActiveDisplayYMinimum=-0.075670313190525529  ActiveDisplayYMaximum=0.68103281871472987  DataLoggingVariableName=ScopeData27
      Scope29 settings: ActiveDisplayYMinimum=-1  ActiveDisplayYMaximum=1  DataLoggingVariableName=ScopeData29
      Scope31 settings: ActiveDisplayYMinimum=-1  ActiveDisplayYMaximum=1  DataLoggingVariableName=ScopeData31
      Scope33 settings: ActiveDisplayYMinimum=-1  ActiveDisplayYMaximum=1  DataLoggingVariableName=ScopeData33
      Scope34 settings: ActiveDisplayYMinimum=-0.0832642866839216  ActiveDisplayYMaximum=1.392456590437777  DataLoggingVariableName=ScopeData34
      Scope36 settings: ActiveDisplayYMinimum=-1  ActiveDisplayYMaximum=1  DataLoggingVariableName=ScopeData36
      Scope38 settings: ActiveDisplayYMinimum=-1  ActiveDisplayYMaximum=1  DataLoggingVariableName=ScopeData38
      Scope4 settings: ActiveDisplayYMinimum=-0.075670313190525529  ActiveDisplayYMaximum=0.68103281871472987  DataLoggingVariableName=ScopeData4
      Scope40 settings: ActiveDisplayYMinimum=-1  ActiveDisplayYMaximum=1  DataLoggingVariableName=ScopeData40
      Scope41 settings: ActiveDisplayYMinimum=-0.11707769671312351  ActiveDisplayYMaximum=2.9872369845712248  DataLoggingVariableName=ScopeData41
      Scope43 settings: ActiveDisplayYMinimum=-1  ActiveDisplayYMaximum=1  DataLoggingVariableName=ScopeData43
      Scope45 settings: ActiveDisplayYMinimum=-1  ActiveDisplayYMaximum=1  DataLoggingVariableName=ScopeData45
      Scope47 settings: ActiveDisplayYMinimum=-1  ActiveDisplayYMaximum=1  DataLoggingVariableName=ScopeData47
      Scope48 settings: ActiveDisplayYMinimum=-0.68698929622800375  ActiveDisplayYMaximum=3.6810932038652076  DataLoggingVariableName=ScopeData48
      Scope50 settings: ActiveDisplayYMinimum=-1  ActiveDisplayYMaximum=1  DataLoggingVariableName=ScopeData50
      Scope52 settings: ActiveDisplayYMinimum=-1  ActiveDisplayYMaximum=1  DataLoggingVariableName=ScopeData52
      Scope54 settings: ActiveDisplayYMinimum=-1  ActiveDisplayYMaximum=1  DataLoggingVariableName=ScopeData54
      Scope55 settings: ActiveDisplayYMinimum=0.64358289012482817  ActiveDisplayYMaximum=1.2950735121479529  DataLoggingVariableName=ScopeData55
      Scope57 settings: ActiveDisplayYMinimum=-1  ActiveDisplayYMaximum=1  DataLoggingVariableName=ScopeData57
      Scope59 settings: ActiveDisplayYMinimum=-1  ActiveDisplayYMaximum=1  DataLoggingVariableName=ScopeData59
      Scope61 settings: ActiveDisplayYMinimum=-1  ActiveDisplayYMaximum=1  DataLoggingVariableName=ScopeData61
      Scope62 settings: ActiveDisplayYMinimum=-0.2530280975880328  ActiveDisplayYMaximum=3.0065023177605332  DataLoggingVariableName=ScopeData62
      Scope64 settings: ActiveDisplayYMinimum=-1  ActiveDisplayYMaximum=1  DataLoggingVariableName=ScopeData64
      Scope66 settings: ActiveDisplayYMinimum=-1  ActiveDisplayYMaximum=1  DataLoggingVariableName=ScopeData66
      Scope68 settings: ActiveDisplayYMinimum=-1  ActiveDisplayYMaximum=1  DataLoggingVariableName=ScopeData68
      Scope69 settings: ActiveDisplayYMinimum=-2.3073793620677803  ActiveDisplayYMaximum=5.5370692283111751  DataLoggingVariableName=ScopeData69
      Scope70 settings: DataLoggingVariableName=ScopeData70
      Scope71 settings: ActiveDisplayYMinimum=-1.7147845226954741  ActiveDisplayYMaximum=10.951620607302841  DataLoggingVariableName=ScopeData71
      Scope72 settings: ActiveDisplayYMinimum=-0.14917696858832405  ActiveDisplayYMaximum=1.3425927172949166  DataLoggingVariableName=ScopeData72
  Scope17 : Scope  NumInputPorts=4
      settings: ActiveDisplayYMinimum=-0.13683516153339964  ActiveDisplayYMaximum=0.88462098401245615  DataLoggingVariableName=ScopeData17
  Scope19 : Scope  NumInputPorts=4
      settings: ActiveDisplayYMinimum=0.033140999285954931  ActiveDisplayYMaximum=0.75907081147207056  DataLoggingVariableName=ScopeData19
  Scope21 : Scope  NumInputPorts=2
      settings: ActiveDisplayYMinimum=-0.27118768326540277  ActiveDisplayYMaximum=1.1954462001960824  DataLoggingVariableName=ScopeData21
  Scope24 : Scope  NumInputPorts=4
      settings: ActiveDisplayYMinimum=-0.53300311339081663  ActiveDisplayYMaximum=5.3830830725693053  DataLoggingVariableName=ScopeData24
  Scope26 : Scope  NumInputPorts=2
      settings: ActiveDisplayYMinimum=-0.18696686921810257  ActiveDisplayYMaximum=0.98227845363936228  DataLoggingVariableName=ScopeData26
  Scope{28,30,32,35,37,39,42,44,46,49,51,53,56,58,60,63,65,67} (18 alike) : Scope  NumInputPorts=3
      Scope28 settings: ActiveDisplayYMinimum=-0.058748502903194777  ActiveDisplayYMaximum=2.8930566334548384  DataLoggingVariableName=ScopeData28
      Scope30 settings: ActiveDisplayYMinimum=-0.058748502903194777  ActiveDisplayYMaximum=2.8930566334548384  DataLoggingVariableName=ScopeData30
      Scope32 settings: ActiveDisplayYMinimum=-0.058748502903194777  ActiveDisplayYMaximum=2.8930566334548384  DataLoggingVariableName=ScopeData32
      Scope35 settings: ActiveDisplayYMinimum=-0.058748502903194777  ActiveDisplayYMaximum=2.8930566334548384  DataLoggingVariableName=ScopeData35
      Scope37 settings: ActiveDisplayYMinimum=-0.058748502903194777  ActiveDisplayYMaximum=2.8930566334548384  DataLoggingVariableName=ScopeData37
      Scope39 settings: ActiveDisplayYMinimum=-0.058748502903194777  ActiveDisplayYMaximum=2.8930566334548384  DataLoggingVariableName=ScopeData39
      Scope42 settings: ActiveDisplayYMinimum=-0.058748502903194777  ActiveDisplayYMaximum=2.8930566334548384  DataLoggingVariableName=ScopeData42
      Scope44 settings: ActiveDisplayYMinimum=-0.058748502903194777  ActiveDisplayYMaximum=2.8930566334548384  DataLoggingVariableName=ScopeData44
      Scope46 settings: ActiveDisplayYMinimum=-0.058748502903194777  ActiveDisplayYMaximum=2.8930566334548384  DataLoggingVariableName=ScopeData46
      Scope49 settings: ActiveDisplayYMinimum=-0.058748502903194777  ActiveDisplayYMaximum=2.8930566334548384  DataLoggingVariableName=ScopeData49
      Scope51 settings: ActiveDisplayYMinimum=-0.058748502903194777  ActiveDisplayYMaximum=2.8930566334548384  DataLoggingVariableName=ScopeData51
      Scope53 settings: ActiveDisplayYMinimum=-0.058748502903194777  ActiveDisplayYMaximum=2.8930566334548384  DataLoggingVariableName=ScopeData53
      Scope56 settings: ActiveDisplayYMinimum=-0.67913635365515379  ActiveDisplayYMaximum=3.4743499013131247  DataLoggingVariableName=ScopeData56
      Scope58 settings: ActiveDisplayYMinimum=0.072085466610230853  ActiveDisplayYMaximum=4.2255717215785111  DataLoggingVariableName=ScopeData58
      Scope60 settings: ActiveDisplayYMinimum=-0.058748502903194777  ActiveDisplayYMaximum=2.8930566334548384  DataLoggingVariableName=ScopeData60
      Scope63 settings: ActiveDisplayYMinimum=-0.058748502903194777  ActiveDisplayYMaximum=2.8930566334548384  DataLoggingVariableName=ScopeData63
      Scope65 settings: ActiveDisplayYMinimum=-0.058748502903194777  ActiveDisplayYMaximum=2.8930566334548384  DataLoggingVariableName=ScopeData65
      Scope67 settings: ActiveDisplayYMinimum=-0.058748502903194777  ActiveDisplayYMaximum=2.8930566334548384  DataLoggingVariableName=ScopeData67
  Scope3 : Scope  NumInputPorts=2
      settings: ActiveDisplayYMinimum=-0.018886009482238258  ActiveDisplayYMaximum=0.33029864219324878  DataLoggingVariableName=ScopeData3
  Simulink-PS Converter : nesl_utility/Simulink-PS Converter  PhysicalDomain=network_engine_domain  SubClassName=ps_input  LeftPortType=input  RightPortType=output  PseudoPeriodic=off  Frequencies=[]  NoiseDistribution=none  NoiseParameters=[]  Unit=V  AffineConversion=off  FilteringAndDerivatives=provide  SimscapeFilterOrder=1  InputFilterTimeConstant=0.001  UdotUserProvided=0
  Simulink-PS Converter1 : nesl_utility/Simulink-PS Converter  PhysicalDomain=network_engine_domain  SubClassName=ps_input  LeftPortType=input  RightPortType=output  PseudoPeriodic=off  Frequencies=[]  NoiseDistribution=none  NoiseParameters=[]  Unit=V  AffineConversion=off  FilteringAndDerivatives=provide  SimscapeFilterOrder=1  InputFilterTimeConstant=0.001  UdotUserProvided=0
  Simulink-PS Converter2 : nesl_utility/Simulink-PS Converter  PhysicalDomain=network_engine_domain  SubClassName=ps_input  LeftPortType=input  RightPortType=output  PseudoPeriodic=off  Frequencies=[]  NoiseDistribution=none  NoiseParameters=[]  Unit=V  AffineConversion=off  FilteringAndDerivatives=provide  SimscapeFilterOrder=1  InputFilterTimeConstant=0.001  UdotUserProvided=0
  Solver Configuration : nesl_utility/Solver Configuration  PhysicalDomain=network_engine_domain  SubClassName=solver  LeftPortType=input  RightPortType=generic  Tones=[]  Harmonics=[]  SimulateNoise=off  Profile=off  UseLocalSampling=off  EnableSwitchedLinearOptims=on  FrequencyDomain=off  UseCCode=off  RelTol=0.001  AbsTol=0.001  MinStep=1e-09  ToWorkspace=off  RevertToSquareIcSolve=off  NumHomotopyIterations=100  PhasorMode=off  PhasorModeNumHarmonics=1  ConsistencySolver=NEWTON_XTOL_AFTER_FTOL  IndexReductionMethod=DerivativeReplacement  DoDC=off  ResidualTolerance=1e-09  ConsistencyTolSource=GLOBAL  ConsistencyAbsTol=0.001  ConsistencyRelTol=0.001  ConsistencyTolFactor=0.001  UseLocalSolver=off  LocalSolverChoice=NE_BACKWARD_EULER_ADVANCER  ResolveIndetEquations=on  FunctionEvalNumThread=1  LocalSolverSampleTime=0.001  DoFixedCost=off  MaxNonlinIter=3  MaxModeIter=2  ComputeImpulses=off  ImpulseIterations=2  LinearAlgebra=auto  LinearAlgebraNumThread=0  EquationFormulation=NE_TIME_EF  DelaysMemoryBudget=1024  AutomaticFiltering=on  FilteringTimeConstant=0.001  PartitionStorageMethod=AS_NEEDED  PartitionMemoryBudget=1024  PartitionMethod=ROBUST  MultibodyUseLocalSolver=off  MultibodyLocalSolverChoice=ODE1  MultibodyLocalSolverSampleTime=0.001
  Solver Configuration1 : nesl_utility/Solver Configuration  PhysicalDomain=network_engine_domain  SubClassName=solver  LeftPortType=input  RightPortType=generic  Tones=[]  Harmonics=[]  SimulateNoise=off  Profile=off  UseLocalSampling=off  EnableSwitchedLinearOptims=on  FrequencyDomain=off  UseCCode=off  RelTol=0.001  AbsTol=0.001  MinStep=1e-09  ToWorkspace=off  RevertToSquareIcSolve=off  NumHomotopyIterations=100  PhasorMode=off  PhasorModeNumHarmonics=1  ConsistencySolver=NEWTON_XTOL_AFTER_FTOL  IndexReductionMethod=DerivativeReplacement  DoDC=off  ResidualTolerance=1e-09  ConsistencyTolSource=GLOBAL  ConsistencyAbsTol=0.001  ConsistencyRelTol=0.001  ConsistencyTolFactor=0.001  UseLocalSolver=off  LocalSolverChoice=NE_BACKWARD_EULER_ADVANCER  ResolveIndetEquations=on  FunctionEvalNumThread=1  LocalSolverSampleTime=0.001  DoFixedCost=off  MaxNonlinIter=3  MaxModeIter=2  ComputeImpulses=off  ImpulseIterations=2  LinearAlgebra=auto  LinearAlgebraNumThread=0  EquationFormulation=NE_TIME_EF  DelaysMemoryBudget=1024  AutomaticFiltering=on  FilteringTimeConstant=0.001  PartitionStorageMethod=AS_NEEDED  PartitionMemoryBudget=1024  PartitionMethod=ROBUST  MultibodyUseLocalSolver=off  MultibodyLocalSolverChoice=ODE1  MultibodyLocalSolverSampleTime=0.001
  Solver Configuration2 : nesl_utility/Solver Configuration  PhysicalDomain=network_engine_domain  SubClassName=solver  LeftPortType=input  RightPortType=generic  Tones=[]  Harmonics=[]  SimulateNoise=off  Profile=off  UseLocalSampling=off  EnableSwitchedLinearOptims=on  FrequencyDomain=off  UseCCode=off  RelTol=0.001  AbsTol=0.001  MinStep=1e-09  ToWorkspace=off  RevertToSquareIcSolve=off  NumHomotopyIterations=100  PhasorMode=off  PhasorModeNumHarmonics=1  ConsistencySolver=NEWTON_XTOL_AFTER_FTOL  IndexReductionMethod=DerivativeReplacement  DoDC=off  ResidualTolerance=1e-09  ConsistencyTolSource=GLOBAL  ConsistencyAbsTol=0.001  ConsistencyRelTol=0.001  ConsistencyTolFactor=0.001  UseLocalSolver=off  LocalSolverChoice=NE_BACKWARD_EULER_ADVANCER  ResolveIndetEquations=on  FunctionEvalNumThread=1  LocalSolverSampleTime=0.001  DoFixedCost=off  MaxNonlinIter=3  MaxModeIter=2  ComputeImpulses=off  ImpulseIterations=2  LinearAlgebra=auto  LinearAlgebraNumThread=0  EquationFormulation=NE_TIME_EF  DelaysMemoryBudget=1024  AutomaticFiltering=on  FilteringTimeConstant=0.001  PartitionStorageMethod=AS_NEEDED  PartitionMemoryBudget=1024  PartitionMethod=ROBUST  MultibodyUseLocalSolver=off  MultibodyLocalSolverChoice=ODE1  MultibodyLocalSolverSampleTime=0.001
  Step{,9..10,17,25} (5 alike) : Step  SampleTime=0
  Step{6,11,13,18,20} (5 alike) : Step  After=2.5  SampleTime=0
  Step{7,14,16,21,23} (5 alike) : Step  After=5  SampleTime=0
  Sum{6..23} (18 alike) : Sum  Inputs=|+-
  Transfer Fcn14 : TransferFcn  Numerator=[0.6075]  Denominator=[1 0]
  Transfer Fcn17 : TransferFcn  Numerator=[0.6075]  Denominator=[1 0]
  Transfer Fcn2 : TransferFcn  Numerator=[33792]  Denominator=[1 2500 55822 0]
  Transfer Fcn4 : TransferFcn  Numerator=[33792]  Denominator=[1 2500 55822 0]
  Transfer Fcn6 : TransferFcn  Numerator=[33792]  Denominator=[1 2500 55822 0]
  Transfer Fcn8 : TransferFcn  Numerator=[0.6075]  Denominator=[1 0]
  Transport Delay : TransportDelay  DelayTime=0.0464
  Transport Delay1 : TransportDelay  DelayTime=0.0464
  Transport Delay2 : TransportDelay  DelayTime=0.0464
  wires:
  PS-Simulink Converter6/1 -> Scope20/1
  Sum13/1 -> Scope47/1, PID Controller13/1
  Transfer Fcn17/1 -> Transport Delay2/1
  PID Controller13/1 -> Cluett y Wang - TCL=4tm2/1
  Step7/1 -> Scope26/2, Simulink-PS Converter2/1, Transfer Fcn14/1, Scope24/4, Transfer Fcn6/1
  Original Function 17/1 -> Scope65/1
  PID Controller7/1 -> Scope70/1, Cluett y Wang - TCL=5tm/1
  PS-Simulink Converter2/1 -> Scope2/1
  Step25/1 -> Scope51/3, Original Function 11/1, Sum21/1
  Sum14/1 -> Scope43/1, PID Controller14/1
  Cluett y Wang - TCL=6tm2/1 -> Mux3/3, Scope42/2, Sum14/2
  Transport Delay1/1 -> Scope24/3
  Mux5/1 -> Scope62/1
  PID Controller12/1 -> Cluett y Wang - TCL=5tm2/1
  Step13/1 -> Scope37/3, Original Function 5/1, Sum10/1
  In1/1 -> Mux1/2, Scope28/3, Original Function 1/1, Sum6/1
  Original Function 6/1 -> Scope39/1
  Step10/1 -> Scope32/3, Original Function 3/1, Sum8/1
  Original Function 4/1 -> Mux2/1, Scope35/1
  Leonard (1994)2/1 -> Mux6/3, Scope63/2, Sum19/2
  Step6/1 -> Scope21/2, Simulink-PS Converter1/1, Transfer Fcn17/1, Scope19/4, Transfer Fcn4/1
  Original Function 13/1 -> Mux5/1, Scope56/1
  Cluett y Wang - TCL=4tm1/1 -> Mux2/5, Scope39/2, Sum11/2
  Step/1 -> Scope3/2, Simulink-PS Converter/1, Transfer Fcn8/1, Scope17/4, Transfer Fcn2/1
  Sum19/1 -> Scope64/1, PID Controller19/1
  Original Function 1/1 -> Mux1/1, Scope28/1
  Original Function 14/1 -> Scope58/1
  Cluett y Wang - TCL=5tm/1 -> Mux1/4, Scope30/2, Sum7/2
  Sum10/1 -> Scope38/1, PID Controller10/1
  In3/1 -> Mux3/2, Scope42/3, Original Function 7/1, Sum14/1
  Original Function 12/1 -> Scope53/1
  Cluett y Wang - TCL=5tm2/1 -> Mux3/4, Scope44/2, Sum12/2
  Transfer Fcn8/1 -> Transport Delay/1
  Step11/1 -> Scope39/3, Original Function 6/1, Sum11/1
  PID Controller14/1 -> Cluett y Wang - TCL=6tm2/1
  Original Function 18/1 -> Scope67/1
  PID Controller8/1 -> Cluett y Wang - TCL=4tm/1
  Mux2/1 -> Scope41/1
  Step17/1 -> Scope53/3, Original Function 12/1, Sum22/1
  PID Controller19/1 -> Leonard (1994)2/1
  PS-Simulink Converter4/1 -> Scope19/1, Scope21/1
  Cluett y Wang - TCL=6tm3/1 -> Mux4/4, Scope51/2, Sum21/2
  PS-Simulink Converter5/1 -> Scope22/1
  Step20/1 -> Scope58/3, Original Function 14/1, Sum15/1
  PID Controller15/1 -> Cluett y Wang - TCL=6tm4/1
  Original Function 8/1 -> Scope44/1
  Original Function 7/1 -> Mux3/1, Scope42/1
  Transport Delay/1 -> Scope17/3
  PID Controller22/1 -> Astrom y Hagglund/1
  Step16/1 -> Scope44/3, Original Function 8/1, Sum12/1
  PID Controller23/1 -> Leonard (1994)1/1
  PID Controller9/1 -> Cluett y Wang - TCL=6tm1/1
  Sum6/1 -> Scope29/1, PID Controller6/1
  Mux4/1 -> Scope55/1
  In5/1 -> Mux5/2, Scope56/3, Original Function 13/1, Sum23/1
  Original Function 2/1 -> Scope30/1
  Sum18/1 -> Scope68/1, PID Controller18/1
  Sum17/1 -> Scope66/1, PID Controller17/1
  Sum20/1 -> Scope50/1, PID Controller20/1
  PID Controller21/1 -> Cluett y Wang - TCL=6tm3/1
  PS-Simulink Converter1/1 -> Scope4/1
  PID Controller6/1 -> Scope71/1, Cluett y Wang - TCL=6tm/1
  PID Controller16/1 -> Astrom y Hagglund1/1
  Original Function 16/1 -> Mux6/1, Scope63/1
  Sum22/1 -> Scope54/1, PID Controller22/1
  PS-Simulink Converter10/1 -> Scope25/1
  Cluett y Wang - TCL=6tm1/1 -> Mux2/3, Scope35/2, Sum9/2
  PS-Simulink Converter7/1 -> Scope18/1
  PID Controller11/1 -> Cluett y Wang - TCL=4tm1/1
  PS-Simulink Converter3/1 -> Scope1/1
  Astrom y Hagglund/1 -> Mux4/5, Scope53/2, Sum22/2
  Transfer Fcn4/1 -> Scope19/2
  Original Function 9/1 -> Scope46/1
  Cluett y Wang - TCL=6tm4/1 -> Mux5/4, Scope58/2, Sum15/2
  PID Controller10/1 -> Cluett y Wang - TCL=5tm1/1
  Leonard (1994)/1 -> Mux4/3, Scope49/2, Sum20/2
  Original Function 3/1 -> Scope32/1
  Sum15/1 -> Scope59/1, PID Controller15/1
  In2/1 -> Mux2/2, Scope35/3, Original Function 4/1, Sum9/1
  Sum21/1 -> Scope52/1, PID Controller21/1
  Original Function 11/1 -> Scope51/1
  Original Function 5/1 -> Scope37/1
  Cluett y Wang - TCL=4tm2/1 -> Mux3/5, Scope46/2, Sum13/2
  PS-Simulink Converter11/1 -> Scope23/1
  PS-Simulink Converter9/1 -> Scope27/1
  Cluett y Wang - TCL=5tm1/1 -> Mux2/4, Scope37/2, Sum10/2
  Astrom y Hagglund2/1 -> Mux6/5, Scope67/2, Sum18/2
  Cluett y Wang - TCL=4tm/1 -> Mux1/5, Scope32/2, Sum8/2
  Transfer Fcn2/1 -> Scope17/2
  Step21/1 -> Scope67/3, Original Function 18/1, Sum18/1
  Step23/1 -> Scope65/3, Original Function 17/1, Sum17/1
  Mux6/1 -> Scope69/1
  Step9/1 -> Scope30/3, Original Function 2/1, Sum7/1
  PID Controller18/1 -> Astrom y Hagglund2/1
  Sum8/1 -> Scope33/1, PID Controller8/1
  Sum23/1 -> Scope57/1, PID Controller23/1
  Cluett y Wang - TCL=6tm/1 -> Mux1/3, Scope28/2, Scope72/1, Sum6/2
  PID Controller17/1 -> Cluett y Wang - TCL=6tm5/1
  Mux3/1 -> Scope48/1
  PID Controller20/1 -> Leonard (1994)/1
  PS-Simulink Converter/1 -> Scope17/1, Scope3/1
  In6/1 -> Mux6/2, Scope63/3, Original Function 16/1, Sum19/1
  Step14/1 -> Scope46/3, Original Function 9/1, Sum13/1
  Original Function 15/1 -> Scope60/1
  Astrom y Hagglund1/1 -> Mux5/5, Scope60/2, Sum16/2
  PS-Simulink Converter8/1 -> Scope24/1, Scope26/1
  Sum7/1 -> Scope31/1, PID Controller7/1
  Original Function 10/1 -> Mux4/1, Scope49/1
  Sum12/1 -> Scope45/1, PID Controller12/1
  Sum16/1 -> Scope61/1, PID Controller16/1
  In4/1 -> Mux4/2, Scope49/3, Original Function 10/1, Sum20/1
  Transport Delay2/1 -> Scope19/3
  Cluett y Wang - TCL=6tm5/1 -> Mux6/4, Scope65/2, Sum17/2
  Mux1/1 -> Scope34/1
  Leonard (1994)1/1 -> Mux5/3, Scope56/2, Sum23/2
  Transfer Fcn14/1 -> Transport Delay1/1
  Sum11/1 -> Scope40/1, PID Controller11/1
  Sum9/1 -> Scope36/1, PID Controller9/1
  Transfer Fcn6/1 -> Scope24/2
  Step18/1 -> Scope60/3, Original Function 15/1, Sum16/1
  connections:
  Rotational Electromechanical Converter/RConn2 -- Mechanical Rotational Reference/LConn1 -- Ideal Rotational Motion Sensor/RConn1 -- Dm/RConn1 -- Solver Configuration/RConn1
  Electrical Reference/LConn1 -- Controlled Voltage Source/RConn2 -- Rotational Electromechanical Converter/RConn1
  Ideal Torque Sensor3/LConn1 -- Gear Box2/RConn1 -- Dm2/LConn1 -- Rotational Electromechanical Converter2/LConn2
  Jl1/LConn1 -- Gear Box1/LConn1 -- Ideal Rotational Motion Sensor1/LConn1
  Rotational Electromechanical Converter/LConn2 -- Dm/LConn1 -- Gear Box/RConn1 -- Ideal Torque Sensor1/LConn1
  Rotational Electromechanical Converter2/RConn2 -- Mechanical Rotational Reference2/LConn1 -- Solver Configuration2/RConn1 -- Ideal Rotational Motion Sensor2/RConn1 -- Dm2/RConn1
  Rotational Electromechanical Converter2/RConn1 -- Electrical Reference2/LConn1 -- Controlled Voltage Source2/RConn2
  Rotational Electromechanical Converter1/RConn2 -- Solver Configuration1/RConn1 -- Ideal Rotational Motion Sensor1/RConn1 -- Dm1/RConn1 -- Mechanical Rotational Reference1/LConn1
  Jl2/LConn1 -- Gear Box2/LConn1 -- Ideal Rotational Motion Sensor2/LConn1
  Gear Box/LConn1 -- Ideal Rotational Motion Sensor/LConn1 -- Jl/LConn1
  Rotational Electromechanical Converter1/RConn1 -- Electrical Reference1/LConn1 -- Controlled Voltage Source1/RConn2
  Gear Box1/RConn1 -- Dm1/LConn1 -- Ideal Torque Sensor2/LConn1 -- Rotational Electromechanical Converter1/LConn2
  Ideal Torque Sensor1/RConn1 -- Jm/LConn1
  Ideal Rotational Motion Sensor/RConn3 -- PS-Simulink Converter/LConn1
  L2/LConn1 -- R2/RConn1
  Ideal Torque Sensor3/RConn2 -- PS-Simulink Converter11/LConn1
  Rotational Electromechanical Converter2/LConn1 -- Current Sensor2/RConn2
  PS-Simulink Converter6/LConn1 -- Ideal Rotational Motion Sensor1/RConn2
  R2/LConn1 -- Controlled Voltage Source2/LConn1
  Ideal Torque Sensor2/RConn2 -- PS-Simulink Converter7/LConn1
  Current Sensor1/LConn1 -- L1/RConn1
  PS-Simulink Converter1/LConn1 -- Current Sensor/RConn1
  Simulink-PS Converter2/RConn1 -- Controlled Voltage Source2/RConn1
  R1/LConn1 -- Controlled Voltage Source1/LConn1
  R/LConn1 -- Controlled Voltage Source/LConn1
  PS-Simulink Converter9/LConn1 -- Current Sensor2/RConn1
  L/LConn1 -- R/RConn1
  Ideal Torque Sensor3/RConn1 -- Jm2/LConn1
  PS-Simulink Converter10/LConn1 -- Ideal Rotational Motion Sensor2/RConn2
  Simulink-PS Converter/RConn1 -- Controlled Voltage Source/RConn1
  Ideal Rotational Motion Sensor2/RConn3 -- PS-Simulink Converter8/LConn1
  L1/LConn1 -- R1/RConn1
  PS-Simulink Converter5/LConn1 -- Current Sensor1/RConn1
  Ideal Torque Sensor1/RConn2 -- PS-Simulink Converter3/LConn1
  Rotational Electromechanical Converter1/LConn1 -- Current Sensor1/RConn2
  Current Sensor2/LConn1 -- L2/RConn1
  Ideal Torque Sensor2/RConn1 -- Jm1/LConn1
  PS-Simulink Converter2/LConn1 -- Ideal Rotational Motion Sensor/RConn2
  Rotational Electromechanical Converter/LConn1 -- Current Sensor/RConn2
  Ideal Rotational Motion Sensor1/RConn3 -- PS-Simulink Converter4/LConn1
  Simulink-PS Converter1/RConn1 -- Controlled Voltage Source1/RConn1
  Current Sensor/LConn1 -- L/RConn1
